simulink model "accController"  (R2022b)
settings: Solver=FixedStepAuto  StartTime=0.0  StopTime=120  FixedStep=tSample  RelTol=1e-3  EnableMultiTasking=on
PreLoadFcn:
  | if exist('tl_preloadfcn','file'), tl_preloadfcn(gcs,'22.1.0.27'); end
PostLoadFcn:
  | if exist('tl_postloadfcn','file'), tl_postloadfcn(gcs,'22.1.0.27'); end
InitFcn:
  | if exist('tlds_init','file'), tlds_init(gcs); end
StartFcn:
  | if exist('tlds_start','file'), tlds_start(gcs); end
StopFcn:
  | if exist('tlds_stop','file'), tlds_stop(gcs); end
model workspace (MAT data in the model file):
  obs_1 = 1
  obs_10 = 1
  obs_11 = 1
  obs_12 = 1
  obs_13 = 1
  obs_14 = 1
  obs_15 = 1
  obs_16 = 1
  obs_17 = 1
  obs_18 = 1
  obs_19 = 1
  obs_2 = 1
  obs_20 = 1
  obs_21 = 1
  obs_22 = 1
  obs_23 = 1
  obs_24 = 1
  obs_25 = 1
  obs_26 = 1
  obs_27 = 1
  obs_28 = 1
  obs_29 = 1
  obs_3 = 1
  obs_30 = 1
  obs_31 = 1
  obs_32 = 1
  obs_4 = 1
  obs_5 = 1
  obs_6 = 1
  obs_7 = 1
  obs_8 = 1
  obs_9 = 1
values from neighbouring files (symbols this model uses):
  pLutAccelMagnitude = [0, 0.1, 0.2, 0.3, 0.4, 0.5, 0.6, 0.7, 0.8, 0.9, 1,                        2.5, 3, 3.5, 4, 4.5, 5, 8, 12, 20]    [start.m]
  pLutAccelnSeverity = [0, 0.005, 0.05, 0.1, 0.15, 0.2, 0.3, 0.4, 0.6, 1, 3,                        5, 10, 17, 24, 32, 45, 60, 75, 100]    [start.m]
  pMaxAccAcceleration = 1.5    [start.m]
  pMaxAccDeacceleration = -1.5    [start.m]
  pMaxOperatingSpeed = 180    [start.m]
  pMinOperatingSpeed = 30    [start.m]
  tSample = 0.01    [start.m]
undefined symbols (not defined in the file or in its folder): Pedal, sigbuilder_block, vehicleDistanceRange
libraries: tllib x7
(part 3 of 5)

== system accController/accController/Subsystem/accController/transformEnum2Seconds ==
  note: Ranges
      |
      | Min time gap in s and m at 80 km/h
      |
      | 2.25 - long (50 m)
      | 1.80 - medium (40 m)
      | 1.35 - short (30 m)
      | 1.15 - extremly short (25 m)
  vehicleDistanceRangeEnum : Inport
  Data Type Conversion : DataTypeConversion  OutDataTypeStr=int8  SaturateOnIntegerOverflow=off  RndMeth=Floor
  Multiport Switch : MultiPortSwitch  DataPortOrder=Specify indices  Inputs=5  DataPortIndices={0,1,2,3}  DataPortForDefault=Additional data port  DiagnosticForDefault=Warning  OutDataTypeStr=Inherit: Inherit via back propagation  SaturateOnIntegerOverflow=off  InputSameDT=off  mask(TL_MultiPortSwitch){data={'output',{'lsb',0.01},'autoscaling',{'mode',0},'date',737980.50352149305}}
      settings: CopyFcn=if exist('copy_tlblock','file')==2,copy_tlblock(gcbh);end  DeleteFcn=if exist('delete_tlblock','file')==2,delete_tlblock(gcbh);end  NameChangeFcn=if exist('rename_tlblock','file')==2,rename_tlblock(gcbh);end  OpenFcn=if exist('tl_open_blockdlg','file')==2,tl_open_blockdlg(gcbh);else,open_system(gcbh,'parameter');end
      mask Help: eval(['if exist(''tl_online_help'',''file'') == 2, tl_online_help(''Topic'',''TL_MultiPortSwitch''),else, web([''jar:file:///'',matlabroot,''/help/toolbox/simulink/help.jar!/slref/' lower(get_param(gcbh,'Blocktype')) '.html''], ''-helpbrowser''),end'])
      mask Display:
      | [x,y] = tlDrawBrandOnBlockIcon(gcbh);
      | plot(x,y);
  extremelyShort : Constant  Value=1.15  mask(TL_Constant){data={'date',737854.52191120374}}
      settings: CopyFcn=if exist('copy_tlblock','file')==2,copy_tlblock(gcbh);end  DeleteFcn=if exist('delete_tlblock','file')==2,delete_tlblock(gcbh);end  NameChangeFcn=if exist('rename_tlblock','file')==2,rename_tlblock(gcbh);end  OpenFcn=if exist('tl_open_blockdlg','file')==2,tl_open_blockdlg(gcbh);else,open_system(gcbh,'parameter');end
      mask Help: eval(['if exist(''tl_online_help'',''file'') == 2, tl_online_help(''Topic'',''TL_Constant''),else, web([''jar:file:///'',matlabroot,''/help/toolbox/simulink/help.jar!/slref/' lower(get_param(gcbh,'Blocktype')) '.html''], ''-helpbrowser''),end'])
      mask Display:
      | [x,y] = tlDrawBrandOnBlockIcon(gcbh);
      | plot(x,y);
  long : Constant  Value=2.25  mask(TL_Constant){data={'date',737854.5230081944}}
      settings: CopyFcn=if exist('copy_tlblock','file')==2,copy_tlblock(gcbh);end  DeleteFcn=if exist('delete_tlblock','file')==2,delete_tlblock(gcbh);end  NameChangeFcn=if exist('rename_tlblock','file')==2,rename_tlblock(gcbh);end  OpenFcn=if exist('tl_open_blockdlg','file')==2,tl_open_blockdlg(gcbh);else,open_system(gcbh,'parameter');end
      mask Help: eval(['if exist(''tl_online_help'',''file'') == 2, tl_online_help(''Topic'',''TL_Constant''),else, web([''jar:file:///'',matlabroot,''/help/toolbox/simulink/help.jar!/slref/' lower(get_param(gcbh,'Blocktype')) '.html''], ''-helpbrowser''),end'])
      mask Display:
      | [x,y] = tlDrawBrandOnBlockIcon(gcbh);
      | plot(x,y);
  medium : Constant  Value=1.8  mask(TL_Constant){data={'date',737854.5223616435}}
      settings: CopyFcn=if exist('copy_tlblock','file')==2,copy_tlblock(gcbh);end  DeleteFcn=if exist('delete_tlblock','file')==2,delete_tlblock(gcbh);end  NameChangeFcn=if exist('rename_tlblock','file')==2,rename_tlblock(gcbh);end  OpenFcn=if exist('tl_open_blockdlg','file')==2,tl_open_blockdlg(gcbh);else,open_system(gcbh,'parameter');end
      mask Help: eval(['if exist(''tl_online_help'',''file'') == 2, tl_online_help(''Topic'',''TL_Constant''),else, web([''jar:file:///'',matlabroot,''/help/toolbox/simulink/help.jar!/slref/' lower(get_param(gcbh,'Blocktype')) '.html''], ''-helpbrowser''),end'])
      mask Display:
      | [x,y] = tlDrawBrandOnBlockIcon(gcbh);
      | plot(x,y);
  short : Constant  Value=1.35  mask(TL_Constant){data={'date',737854.52225954866}}
      settings: CopyFcn=if exist('copy_tlblock','file')==2,copy_tlblock(gcbh);end  DeleteFcn=if exist('delete_tlblock','file')==2,delete_tlblock(gcbh);end  NameChangeFcn=if exist('rename_tlblock','file')==2,rename_tlblock(gcbh);end  OpenFcn=if exist('tl_open_blockdlg','file')==2,tl_open_blockdlg(gcbh);else,open_system(gcbh,'parameter');end
      mask Help: eval(['if exist(''tl_online_help'',''file'') == 2, tl_online_help(''Topic'',''TL_Constant''),else, web([''jar:file:///'',matlabroot,''/help/toolbox/simulink/help.jar!/slref/' lower(get_param(gcbh,'Blocktype')) '.html''], ''-helpbrowser''),end'])
      mask Display:
      | [x,y] = tlDrawBrandOnBlockIcon(gcbh);
      | plot(x,y);
  vehicleDistanceRangeSeconds : Outport
  wires:
  vehicleDistanceRangeEnum/1 -> Data Type Conversion/1
  extremelyShort/1 -> Multiport Switch/5
  long/1 -> Multiport Switch/2
  medium/1 -> Multiport Switch/3
  short/1 -> Multiport Switch/6, Multiport Switch/4
  Multiport Switch/1 -> vehicleDistanceRangeSeconds/1
  Data Type Conversion/1 -> Multiport Switch/1

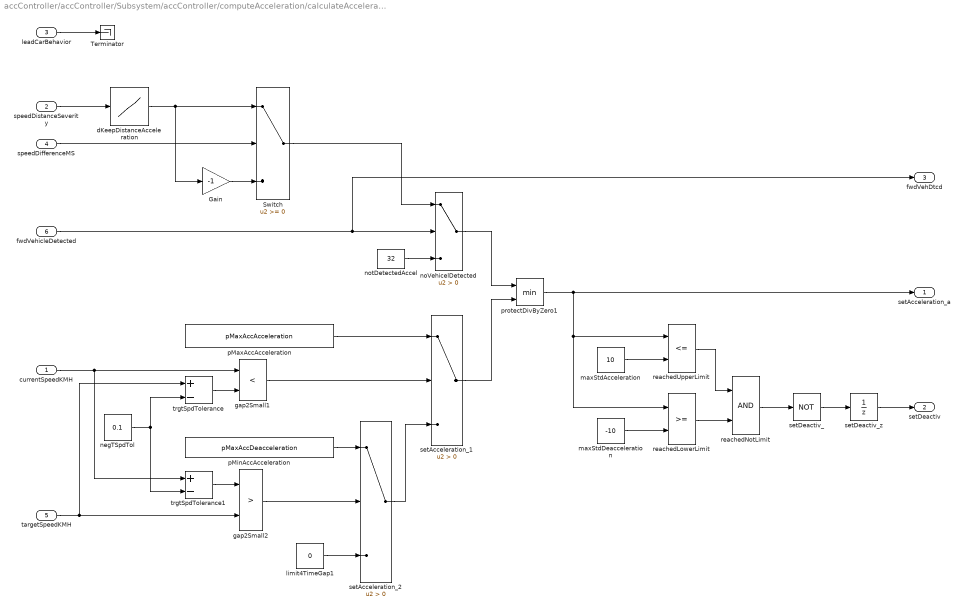
== system accController/accController/Subsystem/accController/computeAcceleration/calculateAcceleration ==
  currentSpeedKMH : Inport
  speedDistanceSeverity : Inport  Port=2
  leadCarBehavior : Inport  Port=3
  speedDifferenceMS : Inport  Port=4
  targetSpeedKMH : Inport  Port=5
  fwdVehicleDetected : Inport  Port=6
  Gain : Gain  Gain=-1  mask(TL_Gain){data={'output',{'type','Int32','scaling','SC_ACCL_FINE'},'date',737877.58934976847}}
      settings: CopyFcn=if exist('copy_tlblock','file')==2,copy_tlblock(gcbh);end  DeleteFcn=if exist('delete_tlblock','file')==2,delete_tlblock(gcbh);end  NameChangeFcn=if exist('rename_tlblock','file')==2,rename_tlblock(gcbh);end  OpenFcn=if exist('tl_open_blockdlg','file')==2,tl_open_blockdlg(gcbh);else,open_system(gcbh,'parameter');end
      mask Help: eval(['if exist(''tl_online_help'',''file'') == 2, tl_online_help(''Topic'',''TL_Gain''),else, web([''jar:file:///'',matlabroot,''/help/toolbox/simulink/help.jar!/slref/' lower(get_param(gcbh,'Blocktype')) '.html''], ''-helpbrowser''),end'])
      mask Display:
      | [x,y] = tlDrawBrandOnBlockIcon(gcbh);
      | plot(x,y);
  Switch : Switch  SaturateOnIntegerOverflow=off  InputSameDT=off  mask(TL_Switch){data={'output',{'type','Int32','scaling','SC_ACCL_FINE'},'date',739002.69656456017}}
      settings: CopyFcn=if exist('copy_tlblock','file')==2,copy_tlblock(gcbh);end  DeleteFcn=if exist('delete_tlblock','file')==2,delete_tlblock(gcbh);end  NameChangeFcn=if exist('rename_tlblock','file')==2,rename_tlblock(gcbh);end  OpenFcn=if exist('tl_open_blockdlg','file')==2,tl_open_blockdlg(gcbh);else,open_system(gcbh,'parameter');end
      mask Help: eval(['if exist(''tl_online_help'',''file'') == 2, tl_online_help(''Topic'',''TL_Switch''),else, web([''jar:file:///'',matlabroot,''/help/toolbox/simulink/help.jar!/slref/' lower(get_param(gcbh,'Blocktype')) '.html''], ''-helpbrowser''),end'])
      mask Display:
      | [x,y] = tlDrawBrandOnBlockIcon(gcbh);
      | plot(x,y);
  Terminator : Terminator
  dKeepDistanceAcceleration : Lookup_n-D  NumberOfTableDimensions=1  BreakpointsForDimension1=pLutAccelnSeverity  BreakpointsForDimension2=[1:3]  IndexSearchMethod=Linear search  Table=pLutAccelMagnitude  InterpMethod=Flat  ExtrapMethod=Clip  DiagnosticForOutOfRangeInput=Warning  InternalRulePriority=Speed  RndMeth=Simplest  mask(TL_Lookup1D){data={'input',{'variable','Parameter/pLutAccelnSeverity'},'output',{'type','Int32','scaling','SC_ACCL_FINE'},'table',{'variable','Parameter/pLutAccelMagnitude'},'date',739002.69656317134}}
      settings: CopyFcn=if exist('copy_tlblock','file')==2,copy_tlblock(gcbh);end  DeleteFcn=if exist('delete_tlblock','file')==2,delete_tlblock(gcbh);end  NameChangeFcn=if exist('rename_tlblock','file')==2,rename_tlblock(gcbh);end  OpenFcn=if exist('tl_open_blockdlg','file')==2,tl_open_blockdlg(gcbh);else,open_system(gcbh,'parameter');end
      mask Help: eval(['if exist(''tl_online_help'',''file'') == 2, tl_online_help(''Topic'',''TL_Lookup1D''),else, web([''jar:file:///'',matlabroot,''/help/toolbox/simulink/help.jar!/slref/' lower(get_param(gcbh,'Blocktype')) '.html''], ''-helpbrowser''),end'])
      mask Display:
      | [x,y] = tlDrawBrandOnBlockIcon(gcbh);
      | plot(x,y);
  gap2Small1 : RelationalOperator  Operator=<  OutDataTypeStr=boolean  InputSameDT=off  mask(TL_RelationalOperator){data={'date',737252.50075726851}}
      settings: CopyFcn=if exist('copy_tlblock','file')==2,copy_tlblock(gcbh);end  DeleteFcn=if exist('delete_tlblock','file')==2,delete_tlblock(gcbh);end  NameChangeFcn=if exist('rename_tlblock','file')==2,rename_tlblock(gcbh);end  OpenFcn=if exist('tl_open_blockdlg','file')==2,tl_open_blockdlg(gcbh);else,open_system(gcbh,'parameter');end
      mask Help: eval(['if exist(''tl_online_help'',''file'') == 2, tl_online_help(''Topic'',''TL_RelationalOperator''),else, web([''jar:file:///'',matlabroot,''/help/toolbox/simulink/help.jar!/slref/' lower(get_param(gcbh,'Blocktype')) '.html''], ''-helpbrowser''),end'])
      mask Display:
      | [x,y] = tlDrawBrandOnBlockIcon(gcbh);
      | plot(x,y);
  gap2Small2 : RelationalOperator  Operator=>  OutDataTypeStr=boolean  InputSameDT=off  mask(TL_RelationalOperator){data={'date',737323.63152983796}}
      settings: CopyFcn=if exist('copy_tlblock','file')==2,copy_tlblock(gcbh);end  DeleteFcn=if exist('delete_tlblock','file')==2,delete_tlblock(gcbh);end  NameChangeFcn=if exist('rename_tlblock','file')==2,rename_tlblock(gcbh);end  OpenFcn=if exist('tl_open_blockdlg','file')==2,tl_open_blockdlg(gcbh);else,open_system(gcbh,'parameter');end
      mask Help: eval(['if exist(''tl_online_help'',''file'') == 2, tl_online_help(''Topic'',''TL_RelationalOperator''),else, web([''jar:file:///'',matlabroot,''/help/toolbox/simulink/help.jar!/slref/' lower(get_param(gcbh,'Blocktype')) '.html''], ''-helpbrowser''),end'])
      mask Display:
      | [x,y] = tlDrawBrandOnBlockIcon(gcbh);
      | plot(x,y);
  limit4TimeGap1 : Constant  Value=0  mask(TL_Constant){data={'date',737323.63099049765}}
      settings: CopyFcn=if exist('copy_tlblock','file')==2,copy_tlblock(gcbh);end  DeleteFcn=if exist('delete_tlblock','file')==2,delete_tlblock(gcbh);end  NameChangeFcn=if exist('rename_tlblock','file')==2,rename_tlblock(gcbh);end  OpenFcn=if exist('tl_open_blockdlg','file')==2,tl_open_blockdlg(gcbh);else,open_system(gcbh,'parameter');end
      mask Help: eval(['if exist(''tl_online_help'',''file'') == 2, tl_online_help(''Topic'',''TL_Constant''),else, web([''jar:file:///'',matlabroot,''/help/toolbox/simulink/help.jar!/slref/' lower(get_param(gcbh,'Blocktype')) '.html''], ''-helpbrowser''),end'])
      mask Display:
      | [x,y] = tlDrawBrandOnBlockIcon(gcbh);
      | plot(x,y);
  maxStdAcceleration : Constant  Value=10  mask(TL_Constant){data={'output',{'class','CONST','type','UInt8','scaling','SC_ACCL'},'date',737875.76841753477}}
      settings: CopyFcn=if exist('copy_tlblock','file')==2,copy_tlblock(gcbh);end  DeleteFcn=if exist('delete_tlblock','file')==2,delete_tlblock(gcbh);end  NameChangeFcn=if exist('rename_tlblock','file')==2,rename_tlblock(gcbh);end  OpenFcn=if exist('tl_open_blockdlg','file')==2,tl_open_blockdlg(gcbh);else,open_system(gcbh,'parameter');end
      mask Help: eval(['if exist(''tl_online_help'',''file'') == 2, tl_online_help(''Topic'',''TL_Constant''),else, web([''jar:file:///'',matlabroot,''/help/toolbox/simulink/help.jar!/slref/' lower(get_param(gcbh,'Blocktype')) '.html''], ''-helpbrowser''),end'])
      mask Display:
      | [x,y] = tlDrawBrandOnBlockIcon(gcbh);
      | plot(x,y);
  "maxStdDeacceleration " : Constant  Value=-10  mask(TL_Constant){data={'output',{'class','CONST','type','Int8','scaling','SC_ACCL'},'date',737875.76914055552}}
      settings: CopyFcn=if exist('copy_tlblock','file')==2,copy_tlblock(gcbh);end  DeleteFcn=if exist('delete_tlblock','file')==2,delete_tlblock(gcbh);end  NameChangeFcn=if exist('rename_tlblock','file')==2,rename_tlblock(gcbh);end  OpenFcn=if exist('tl_open_blockdlg','file')==2,tl_open_blockdlg(gcbh);else,open_system(gcbh,'parameter');end
      mask Help: eval(['if exist(''tl_online_help'',''file'') == 2, tl_online_help(''Topic'',''TL_Constant''),else, web([''jar:file:///'',matlabroot,''/help/toolbox/simulink/help.jar!/slref/' lower(get_param(gcbh,'Blocktype')) '.html''], ''-helpbrowser''),end'])
      mask Display:
      | [x,y] = tlDrawBrandOnBlockIcon(gcbh);
      | plot(x,y);
  negTSpdTol : Constant  Value=0.1  mask(TL_Constant){data={'output',{'class','CONST','type','Int32','scaling','SC_ACCL_FINE'},'date',737931.43492643523}}
      settings: CopyFcn=if exist('copy_tlblock','file')==2,copy_tlblock(gcbh);end  DeleteFcn=if exist('delete_tlblock','file')==2,delete_tlblock(gcbh);end  NameChangeFcn=if exist('rename_tlblock','file')==2,rename_tlblock(gcbh);end  OpenFcn=if exist('tl_open_blockdlg','file')==2,tl_open_blockdlg(gcbh);else,open_system(gcbh,'parameter');end
      mask Help: eval(['if exist(''tl_online_help'',''file'') == 2, tl_online_help(''Topic'',''TL_Constant''),else, web([''jar:file:///'',matlabroot,''/help/toolbox/simulink/help.jar!/slref/' lower(get_param(gcbh,'Blocktype')) '.html''], ''-helpbrowser''),end'])
      mask Display:
      | [x,y] = tlDrawBrandOnBlockIcon(gcbh);
      | plot(x,y);
  noVehicelDetected : Switch  Criteria=u2 > Threshold  SaturateOnIntegerOverflow=off  InputSameDT=off  mask(TL_Switch){data={'output',{'name','$D','type','Int32','scaling','SC_ACCL_FINE'},'date',739002.69656468753}}
      settings: CopyFcn=if exist('copy_tlblock','file')==2,copy_tlblock(gcbh);end  DeleteFcn=if exist('delete_tlblock','file')==2,delete_tlblock(gcbh);end  NameChangeFcn=if exist('rename_tlblock','file')==2,rename_tlblock(gcbh);end  OpenFcn=if exist('tl_open_blockdlg','file')==2,tl_open_blockdlg(gcbh);else,open_system(gcbh,'parameter');end
      mask Help: eval(['if exist(''tl_online_help'',''file'') == 2, tl_online_help(''Topic'',''TL_Switch''),else, web([''jar:file:///'',matlabroot,''/help/toolbox/simulink/help.jar!/slref/' lower(get_param(gcbh,'Blocktype')) '.html''], ''-helpbrowser''),end'])
      mask Display:
      | [x,y] = tlDrawBrandOnBlockIcon(gcbh);
      | plot(x,y);
  notDetectedAccel : Constant  Value=32  mask(TL_Constant){data={'output',{'type','Int8'},'date',737841.59936543985}}
      settings: CopyFcn=if exist('copy_tlblock','file')==2,copy_tlblock(gcbh);end  DeleteFcn=if exist('delete_tlblock','file')==2,delete_tlblock(gcbh);end  NameChangeFcn=if exist('rename_tlblock','file')==2,rename_tlblock(gcbh);end  OpenFcn=if exist('tl_open_blockdlg','file')==2,tl_open_blockdlg(gcbh);else,open_system(gcbh,'parameter');end
      mask Help: eval(['if exist(''tl_online_help'',''file'') == 2, tl_online_help(''Topic'',''TL_Constant''),else, web([''jar:file:///'',matlabroot,''/help/toolbox/simulink/help.jar!/slref/' lower(get_param(gcbh,'Blocktype')) '.html''], ''-helpbrowser''),end'])
      mask Display:
      | [x,y] = tlDrawBrandOnBlockIcon(gcbh);
      | plot(x,y);
  pMaxAccAcceleration : Constant  Value=pMaxAccAcceleration  mask(TL_Constant){data={'output',{'variable','Parameter/pMaxAccAcceleration'},'date',737854.50936554396}}
      settings: CopyFcn=if exist('copy_tlblock','file')==2,copy_tlblock(gcbh);end  DeleteFcn=if exist('delete_tlblock','file')==2,delete_tlblock(gcbh);end  NameChangeFcn=if exist('rename_tlblock','file')==2,rename_tlblock(gcbh);end  OpenFcn=if exist('tl_open_blockdlg','file')==2,tl_open_blockdlg(gcbh);else,open_system(gcbh,'parameter');end
      mask Help: eval(['if exist(''tl_online_help'',''file'') == 2, tl_online_help(''Topic'',''TL_Constant''),else, web([''jar:file:///'',matlabroot,''/help/toolbox/simulink/help.jar!/slref/' lower(get_param(gcbh,'Blocktype')) '.html''], ''-helpbrowser''),end'])
      mask Display:
      | [x,y] = tlDrawBrandOnBlockIcon(gcbh);
      | plot(x,y);
  pMinAccAcceleration : Constant  Value=pMaxAccDeacceleration  mask(TL_Constant){data={'output',{'variable','Parameter/pMaxAccDeacceleration'},'date',737925.64861562499}}
      settings: CopyFcn=if exist('copy_tlblock','file')==2,copy_tlblock(gcbh);end  DeleteFcn=if exist('delete_tlblock','file')==2,delete_tlblock(gcbh);end  NameChangeFcn=if exist('rename_tlblock','file')==2,rename_tlblock(gcbh);end  OpenFcn=if exist('tl_open_blockdlg','file')==2,tl_open_blockdlg(gcbh);else,open_system(gcbh,'parameter');end
      mask Help: eval(['if exist(''tl_online_help'',''file'') == 2, tl_online_help(''Topic'',''TL_Constant''),else, web([''jar:file:///'',matlabroot,''/help/toolbox/simulink/help.jar!/slref/' lower(get_param(gcbh,'Blocktype')) '.html''], ''-helpbrowser''),end'])
      mask Display:
      | [x,y] = tlDrawBrandOnBlockIcon(gcbh);
      | plot(x,y);
  protectDivByZero1 : MinMax  Inputs=2  mask(TL_MinMax){data={'output',{'type','Int32','scaling','SC_ACCL_FINE'},'date',739002.69656333339}}
      settings: CopyFcn=if exist('copy_tlblock','file')==2,copy_tlblock(gcbh);end  DeleteFcn=if exist('delete_tlblock','file')==2,delete_tlblock(gcbh);end  NameChangeFcn=if exist('rename_tlblock','file')==2,rename_tlblock(gcbh);end  OpenFcn=if exist('tl_open_blockdlg','file')==2,tl_open_blockdlg(gcbh);else,open_system(gcbh,'parameter');end
      mask Help: eval(['if exist(''tl_online_help'',''file'') == 2, tl_online_help(''Topic'',''TL_MinMax''),else, web([''jar:file:///'',matlabroot,''/help/toolbox/simulink/help.jar!/slref/' lower(get_param(gcbh,'Blocktype')) '.html''], ''-helpbrowser''),end'])
      mask Display:
      | [x,y] = tlDrawBrandOnBlockIcon(gcbh);
      | plot(x,y);
  reachedLowerLimit : RelationalOperator  OutDataTypeStr=boolean  InputSameDT=off  mask(TL_RelationalOperator){data={'date',737252.5420665394}}
      settings: CopyFcn=if exist('copy_tlblock','file')==2,copy_tlblock(gcbh);end  DeleteFcn=if exist('delete_tlblock','file')==2,delete_tlblock(gcbh);end  NameChangeFcn=if exist('rename_tlblock','file')==2,rename_tlblock(gcbh);end  OpenFcn=if exist('tl_open_blockdlg','file')==2,tl_open_blockdlg(gcbh);else,open_system(gcbh,'parameter');end
      mask Help: eval(['if exist(''tl_online_help'',''file'') == 2, tl_online_help(''Topic'',''TL_RelationalOperator''),else, web([''jar:file:///'',matlabroot,''/help/toolbox/simulink/help.jar!/slref/' lower(get_param(gcbh,'Blocktype')) '.html''], ''-helpbrowser''),end'])
      mask Display:
      | [x,y] = tlDrawBrandOnBlockIcon(gcbh);
      | plot(x,y);
  reachedNotLimit : Logic  AllPortsSameDT=off  OutDataTypeStr=boolean  mask(TL_LogicalOperator){data={'date',737252.42547131947}}
      settings: CopyFcn=if exist('copy_tlblock','file')==2,copy_tlblock(gcbh);end  DeleteFcn=if exist('delete_tlblock','file')==2,delete_tlblock(gcbh);end  NameChangeFcn=if exist('rename_tlblock','file')==2,rename_tlblock(gcbh);end  OpenFcn=if exist('tl_open_blockdlg','file')==2,tl_open_blockdlg(gcbh);else,open_system(gcbh,'parameter');end
      mask Help: eval(['if exist(''tl_online_help'',''file'') == 2, tl_online_help(''Topic'',''TL_LogicalOperator''),else, web([''jar:file:///'',matlabroot,''/help/toolbox/simulink/help.jar!/slref/' lower(get_param(gcbh,'Blocktype')) '.html''], ''-helpbrowser''),end'])
      mask Display:
      | [x,y] = tlDrawBrandOnBlockIcon(gcbh);
      | plot(x,y);
  reachedUpperLimit : RelationalOperator  Operator=<=  OutDataTypeStr=boolean  InputSameDT=off  mask(TL_RelationalOperator){data={'date',737252.54271625006}}
      settings: CopyFcn=if exist('copy_tlblock','file')==2,copy_tlblock(gcbh);end  DeleteFcn=if exist('delete_tlblock','file')==2,delete_tlblock(gcbh);end  NameChangeFcn=if exist('rename_tlblock','file')==2,rename_tlblock(gcbh);end  OpenFcn=if exist('tl_open_blockdlg','file')==2,tl_open_blockdlg(gcbh);else,open_system(gcbh,'parameter');end
      mask Help: eval(['if exist(''tl_online_help'',''file'') == 2, tl_online_help(''Topic'',''TL_RelationalOperator''),else, web([''jar:file:///'',matlabroot,''/help/toolbox/simulink/help.jar!/slref/' lower(get_param(gcbh,'Blocktype')) '.html''], ''-helpbrowser''),end'])
      mask Display:
      | [x,y] = tlDrawBrandOnBlockIcon(gcbh);
      | plot(x,y);
  setAcceleration_1 : Switch  Criteria=u2 > Threshold  SaturateOnIntegerOverflow=off  InputSameDT=off  mask(TL_Switch){data={'output',{'type','Int32','scaling','SC_ACCL_FINE'},'date',737930.72515679395}}
      settings: CopyFcn=if exist('copy_tlblock','file')==2,copy_tlblock(gcbh);end  DeleteFcn=if exist('delete_tlblock','file')==2,delete_tlblock(gcbh);end  NameChangeFcn=if exist('rename_tlblock','file')==2,rename_tlblock(gcbh);end  OpenFcn=if exist('tl_open_blockdlg','file')==2,tl_open_blockdlg(gcbh);else,open_system(gcbh,'parameter');end
      mask Help: eval(['if exist(''tl_online_help'',''file'') == 2, tl_online_help(''Topic'',''TL_Switch''),else, web([''jar:file:///'',matlabroot,''/help/toolbox/simulink/help.jar!/slref/' lower(get_param(gcbh,'Blocktype')) '.html''], ''-helpbrowser''),end'])
      mask Display:
      | [x,y] = tlDrawBrandOnBlockIcon(gcbh);
      | plot(x,y);
  setAcceleration_2 : Switch  Criteria=u2 > Threshold  SaturateOnIntegerOverflow=off  InputSameDT=off  mask(TL_Switch){data={'output',{'type','Int32','scaling','SC_ACCL_FINE'},'date',737930.72525260411}}
      settings: CopyFcn=if exist('copy_tlblock','file')==2,copy_tlblock(gcbh);end  DeleteFcn=if exist('delete_tlblock','file')==2,delete_tlblock(gcbh);end  NameChangeFcn=if exist('rename_tlblock','file')==2,rename_tlblock(gcbh);end  OpenFcn=if exist('tl_open_blockdlg','file')==2,tl_open_blockdlg(gcbh);else,open_system(gcbh,'parameter');end
      mask Help: eval(['if exist(''tl_online_help'',''file'') == 2, tl_online_help(''Topic'',''TL_Switch''),else, web([''jar:file:///'',matlabroot,''/help/toolbox/simulink/help.jar!/slref/' lower(get_param(gcbh,'Blocktype')) '.html''], ''-helpbrowser''),end'])
      mask Display:
      | [x,y] = tlDrawBrandOnBlockIcon(gcbh);
      | plot(x,y);
  setDeactiv_ : Logic  Operator=NOT  Inputs=1  AllPortsSameDT=off  OutDataTypeStr=boolean  mask(TL_LogicalOperator){data={'date',737253.49977399304}}
      settings: CopyFcn=if exist('copy_tlblock','file')==2,copy_tlblock(gcbh);end  DeleteFcn=if exist('delete_tlblock','file')==2,delete_tlblock(gcbh);end  NameChangeFcn=if exist('rename_tlblock','file')==2,rename_tlblock(gcbh);end  OpenFcn=if exist('tl_open_blockdlg','file')==2,tl_open_blockdlg(gcbh);else,open_system(gcbh,'parameter');end
      mask Help: eval(['if exist(''tl_online_help'',''file'') == 2, tl_online_help(''Topic'',''TL_LogicalOperator''),else, web([''jar:file:///'',matlabroot,''/help/toolbox/simulink/help.jar!/slref/' lower(get_param(gcbh,'Blocktype')) '.html''], ''-helpbrowser''),end'])
      mask Display:
      | [x,y] = tlDrawBrandOnBlockIcon(gcbh);
      | plot(x,y);
  setDeactiv_z : UnitDelay  SampleTime=-1  HasFrameUpgradeWarning=on  mask(TL_UnitDelay){data={'output',{'type','Bool'},'state',{'type','Bool'},'date',737925.62841307872}}
      settings: AttributesFormatString=Init: %<X0>  CopyFcn=if exist('copy_tlblock','file')==2,copy_tlblock(gcbh);end  DeleteFcn=if exist('delete_tlblock','file')==2,delete_tlblock(gcbh);end  NameChangeFcn=if exist('rename_tlblock','file')==2,rename_tlblock(gcbh);end  OpenFcn=if exist('tl_open_blockdlg','file')==2,tl_open_blockdlg(gcbh);else,open_system(gcbh,'parameter');end
      mask Help: eval(['if exist(''tl_online_help'',''file'') == 2, tl_online_help(''Topic'',''TL_UnitDelay''),else, web([''jar:file:///'',matlabroot,''/help/toolbox/simulink/help.jar!/slref/' lower(get_param(gcbh,'Blocktype')) '.html''], ''-helpbrowser''),end'])
      mask Display:
      | [x,y] = tlDrawBrandOnBlockIcon(gcbh);
      | plot(x,y);
  trgtSpdTolerance : Sum  Inputs=+-  mask(TL_Sum){data={'output',{'type','Int32','scaling','SC_ACCL_FINE'},'date',737931.43510854163}}
      settings: CopyFcn=if exist('copy_tlblock','file')==2,copy_tlblock(gcbh);end  DeleteFcn=if exist('delete_tlblock','file')==2,delete_tlblock(gcbh);end  NameChangeFcn=if exist('rename_tlblock','file')==2,rename_tlblock(gcbh);end  OpenFcn=if exist('tl_open_blockdlg','file')==2,tl_open_blockdlg(gcbh);else,open_system(gcbh,'parameter');end
      mask Help: eval(['if exist(''tl_online_help'',''file'') == 2, tl_online_help(''Topic'',''TL_Sum''),else, web([''jar:file:///'',matlabroot,''/help/toolbox/simulink/help.jar!/slref/' lower(get_param(gcbh,'Blocktype')) '.html''], ''-helpbrowser''),end'])
      mask Display:
      | [x,y] = tlDrawBrandOnBlockIcon(gcbh);
      | plot(x,y);
  trgtSpdTolerance1 : Sum  Inputs=+-  mask(TL_Sum){data={'output',{'type','Int32','scaling','SC_ACCL_FINE'},'date',737931.43525296298}}
      settings: CopyFcn=if exist('copy_tlblock','file')==2,copy_tlblock(gcbh);end  DeleteFcn=if exist('delete_tlblock','file')==2,delete_tlblock(gcbh);end  NameChangeFcn=if exist('rename_tlblock','file')==2,rename_tlblock(gcbh);end  OpenFcn=if exist('tl_open_blockdlg','file')==2,tl_open_blockdlg(gcbh);else,open_system(gcbh,'parameter');end
      mask Help: eval(['if exist(''tl_online_help'',''file'') == 2, tl_online_help(''Topic'',''TL_Sum''),else, web([''jar:file:///'',matlabroot,''/help/toolbox/simulink/help.jar!/slref/' lower(get_param(gcbh,'Blocktype')) '.html''], ''-helpbrowser''),end'])
      mask Display:
      | [x,y] = tlDrawBrandOnBlockIcon(gcbh);
      | plot(x,y);
  setAcceleration_a : Outport
  setDeactiv : Outport  Port=2
  fwdVehDtcd : Outport  Port=3
  wires:
  currentSpeedKMH/1 -> trgtSpdTolerance1/1, gap2Small1/1
  pMaxAccAcceleration/1 -> setAcceleration_1/1
  gap2Small1/1 -> setAcceleration_1/2
  setAcceleration_2/1 -> setAcceleration_1/3
  pMinAccAcceleration/1 -> setAcceleration_2/1
  gap2Small2/1 -> setAcceleration_2/2
  targetSpeedKMH/1 -> trgtSpdTolerance/1, gap2Small2/2
  limit4TimeGap1/1 -> setAcceleration_2/3
  speedDistanceSeverity/1 -> dKeepDistanceAcceleration/1
  fwdVehicleDetected/1 -> fwdVehDtcd/1, noVehicelDetected/2
  notDetectedAccel/1 -> noVehicelDetected/3
  setAcceleration_1/1 -> protectDivByZero1/2
  speedDifferenceMS/1 -> Switch/2
  dKeepDistanceAcceleration/1 -> Gain/1, Switch/1
  Gain/1 -> Switch/3
  Switch/1 -> noVehicelDetected/1
  noVehicelDetected/1 -> protectDivByZero1/1
  protectDivByZero1/1 -> setAcceleration_a/1, reachedLowerLimit/1, reachedUpperLimit/1
  "maxStdDeacceleration "/1 -> reachedLowerLimit/2
  reachedLowerLimit/1 -> reachedNotLimit/2
  maxStdAcceleration/1 -> reachedUpperLimit/2
  reachedUpperLimit/1 -> reachedNotLimit/1
  reachedNotLimit/1 -> setDeactiv_/1
  setDeactiv_/1 -> setDeactiv_z/1
  setDeactiv_z/1 -> setDeactiv/1
  trgtSpdTolerance/1 -> gap2Small1/2
  trgtSpdTolerance1/1 -> gap2Small2/1
  negTSpdTol/1 -> trgtSpdTolerance1/2, trgtSpdTolerance/2
  leadCarBehavior/1 -> Terminator/1

== system accController/accController/Subsystem/accController/computeAcceleration/calculateMinimumDistances ==
  vehicleDistanceRange : Inport
  currentSpeedMeter : Inport  Port=2
  minDistanceMeter : Product  Inputs=**  RndMeth=Zero  mask(TL_Product){data={'output',{'type','Int32','scaling','SC_ACCL_FINE'},'date',737925.64559052081}}
      settings: CopyFcn=if exist('copy_tlblock','file')==2,copy_tlblock(gcbh);end  DeleteFcn=if exist('delete_tlblock','file')==2,delete_tlblock(gcbh);end  NameChangeFcn=if exist('rename_tlblock','file')==2,rename_tlblock(gcbh);end  OpenFcn=if exist('tl_open_blockdlg','file')==2,tl_open_blockdlg(gcbh);else,open_system(gcbh,'parameter');end
      mask Help: eval(['if exist(''tl_online_help'',''file'') == 2, tl_online_help(''Topic'',''TL_Product''),else, web([''jar:file:///'',matlabroot,''/help/toolbox/simulink/help.jar!/slref/' lower(get_param(gcbh,'Blocktype')) '.html''], ''-helpbrowser''),end'])
      mask Display:
      | [x,y] = tlDrawBrandOnBlockIcon(gcbh);
      | plot(x,y);
  "currentMinDistanceMeter " : Outport
  currentMinDistanceSeconds : Outport  Port=2
  wires:
  currentSpeedMeter/1 -> minDistanceMeter/1
  vehicleDistanceRange/1 -> currentMinDistanceSeconds/1, minDistanceMeter/2
  minDistanceMeter/1 -> "currentMinDistanceMeter "/1
